simulink model "DualEncoder"  (R2013a)
settings: Solver=ode45  StartTime=0.0  StopTime=10.0  RelTol=1e-3
libraries: CSLlib x2
settings Model: Creator=Carion  LastModifiedBy=Carion

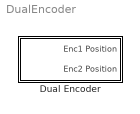
== system DualEncoder ==
  Dual Encoder : Subsystem

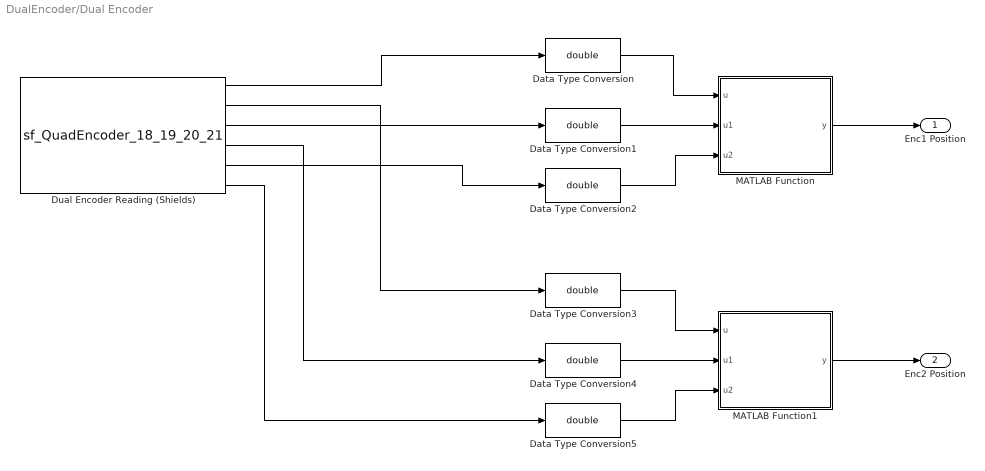
== system DualEncoder/Dual Encoder ==
  Data Type Conversion{,1..5} (6 alike) : DataTypeConversion  OutDataTypeStr=double
  Dual Encoder Reading (Shields) : S-Function  InitFcn=try, set_param(gcb,'FunctionName','sf_QuadEncoder_18_19_20_21'), end  FunctionName=sf_QuadEncoder_18_19_20_21  Parameters=uint8([0 1]),uint8([18 20]),uint8([19 21])  SFunctionModules=sf_QuadEncoder_18_19_20_21_wrapper  EnableBusSupport=off  mask(S-Function Builder){}
      mask init:
      | val = [[.9  0.75 0.75 1 1 .9 .9 1]',[1 1 0.75 0.75 .9 .9 1 .9]'];try , sys = get_param(gcb,'SfunBuilderFcnName');if isempty(sys), sys = get_param(gcb,'FunctionName'); end,catch, sys = get_param(gcb,'FunctionName'); end
      settings: CopyFcn=set_param(gcbh,'LinkStatus','none')  PreSaveFcn=try, set_param(gcb,'FunctionName','sf_QuadEncoder_18_19_20_21'), end  OpenFcn=sfunctionwizard(gcbh)
      mask Display: plot(val(:,1),val(:,2)),disp(sys), port_label('output',1,'pos1'), port_label('output',2,'pos2'), port_label('output',3,'OF1'), port_label('output',4,'OF2'), port_label('output',5,'UF1'), port_label('output',6,'UF2')
  MATLAB Function : Subsystem  TreatAsAtomicUnit=on
  MATLAB Function1 : Subsystem  TreatAsAtomicUnit=on
  Enc1 Position : Outport
  Enc2 Position : Outport  Port=2
  wires:
  Dual Encoder Reading (Shields)/1 -> Data Type Conversion/1
  Dual Encoder Reading (Shields)/2 -> Data Type Conversion3/1
  Dual Encoder Reading (Shields)/3 -> Data Type Conversion1/1
  Dual Encoder Reading (Shields)/4 -> Data Type Conversion4/1
  Dual Encoder Reading (Shields)/5 -> Data Type Conversion2/1
  Dual Encoder Reading (Shields)/6 -> Data Type Conversion5/1
  Data Type Conversion/1 -> MATLAB Function/1(u)
  Data Type Conversion1/1 -> MATLAB Function/2(u1)
  Data Type Conversion2/1 -> MATLAB Function/3(u2)
  Data Type Conversion3/1 -> MATLAB Function1/1(u)
  Data Type Conversion4/1 -> MATLAB Function1/2(u1)
  Data Type Conversion5/1 -> MATLAB Function1/3(u2)
  MATLAB Function/1(y) -> Enc1 Position/1
  MATLAB Function1/1(y) -> Enc2 Position/1

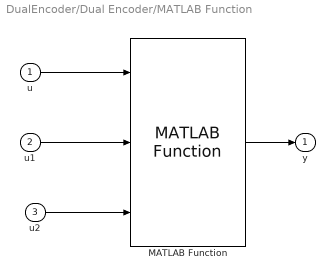
== system DualEncoder/Dual Encoder/MATLAB Function ==
  u : Inport
  u1 : Inport  Port=2
  u2 : Inport  Port=3
  MATLAB Function : CSLlib/QuadEncoder/MATLAB Function
  y : Outport
  wires:
  u/1 -> MATLAB Function/1
  u2/1 -> MATLAB Function/3
  u1/1 -> MATLAB Function/2
  MATLAB Function/1 -> y/1

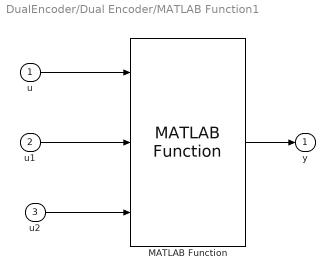
== system DualEncoder/Dual Encoder/MATLAB Function1 ==
  u : Inport
  u1 : Inport  Port=2
  u2 : Inport  Port=3
  MATLAB Function : CSLlib/QuadEncoder/MATLAB Function
  y : Outport
  wires:
  u/1 -> MATLAB Function/1
  u2/1 -> MATLAB Function/3
  u1/1 -> MATLAB Function/2
  MATLAB Function/1 -> y/1
